simulink model "DC_Charging_Sequence_Block_updated"  (R2024b)
settings: Solver=FixedStepDiscrete  StartTime=0.0  StopTime=10.0  FixedStep=0.01  RelTol=1e-3
undefined symbols (not defined in the file or in its folder): CCM, raptor_get_safe_string, raptor_xcp_function
libraries: Raptor_lib x28
settings Model: RaptorUIDSize=4  Raptor_Target=CCM-58NN-112-2403  Raptor_Calloc=NonVolatile (EEPROM)  Raptor_ecuaddr=11  RaptorBuildNum=-1  Creator=noahm  LastModifiedBy=malul
settings OptimizationCC: DefaultParameterBehavior=Inlined  UseSpecifiedMinMax=on  InlineInvariantSignals=on  EnhancedBackFolding=on  PassReuseOutputArgsAs=Individual arguments  InitFltsAndDblsToZero=on  NoFixptDivByZeroProtection=on  EfficientFloat2IntCast=on  OptimizeBlockOrder=speed  DifferentSizesBufferReuse=on  OptimizationCustomize=off  EfficientTunableParamExpr=on
settings DebuggingCC: UnderspecifiedInitializationDetection=Classic  MergeDetectMultiDrivingBlocksExec=none  InheritedTsInSrcMsg=none  ParameterTunabilityLossMsg=error
settings HardwareCC: TargetIntDivRoundTo=Zero  TargetEndianess=BigEndian  ProdEqTarget=off
settings ModelReferenceCC: PropagateSignalLabelsOutOfModel=off
settings SFSimCC: MATLABDynamicMemAlloc=off
settings RTWCC: Description=Raptor (tm)  SystemTargetFile=raptor.tlc  MakeCommand=raptor_make_rtw  TemplateMakefile=raptor_tmf
settings CodeAppCC: ForceParamTrailComments=on  IgnoreCustomStorageClasses=off  MaxIdLength=100  OperatorAnnotations=on  SimulinkDataObjDesc=on  SFDataObjDesc=on  InsertBlockDesc=on
settings STFCustomTargetCC: TargetLangStandard=C99 (ISO)  MultiwordLength=256  GenerateSampleERTMain=on  CombineOutputUpdateFcns=on  CombineSignalStateStructs=on  ERTCustomFileBanners=on  SupportComplex=off  SupportContinuousTime=off  SupportNonInlinedSFcns=off  RemoveResetFunc=on  MATLABClassNameForMDSCustomization=Simulink.SoftwareTarget.ERTCustomization  SystemTargetFile=raptor.tlc
settings ERTTargetCC: TargetLangStandard=C99 (ISO)  GenerateSampleERTMain=on  ParMdlRefBuildCompliant=off  CompOptLevelCompliant=off  ConcurrentExecutionCompliant=off  CombineSignalStateStructs=on  SupportComplex=off  ModelStepFunctionPrototypeControlCompliant=off  CPPClassGenCompliant=off  UseToolchainInfoCompliant=off  ERTCustomFileTemplate=example_file_process.tlc

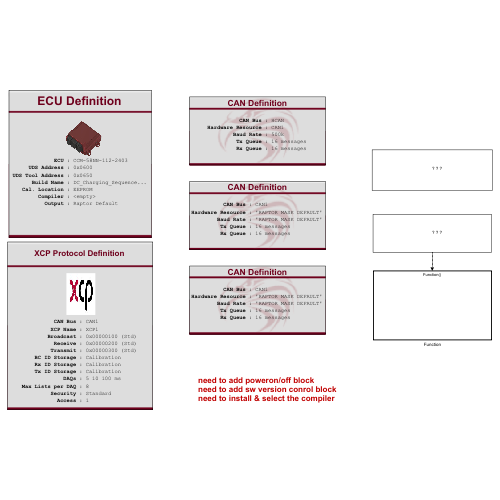
[thumbnail: Simulink's stored preview of the top-level diagram]
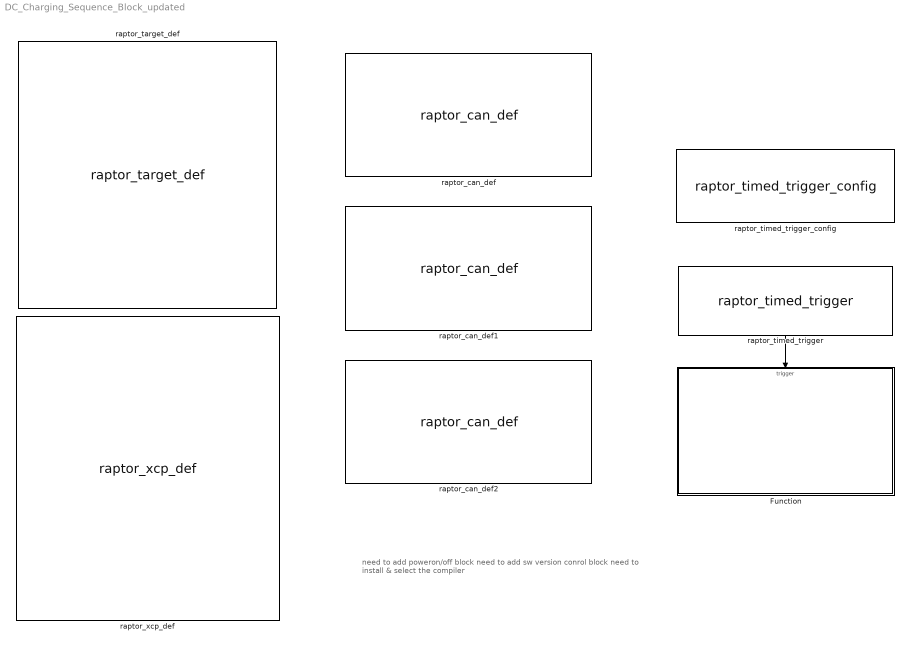
== system DC_Charging_Sequence_Block_updated ==
  note: need to add poweron/off block
      | need to add sw version conrol block
      | need to install & select the compiler
  Function : Subsystem
  raptor_can_def : Raptor_lib/CAN/raptor_can_def  canBus='HCAN'  resourceValues=CAN1|CAN2|CAN3|CAN4|CAN5|CAN6|CAN7|CAN8|(None)  resource=CAN1  baudRateValues=33k|50k|100k|125k|200k|250k|333k|500k|667k|800k|1000k  baudRate=500k  useCustomBR=0  customBR='CustomBaudRate'  enable_baud_rate_config=0  sim_func_name='ConfigureCANBaudRate'  createButton=0  updateButton=0  txQueueSize=16  rxQueueSize=16
      settings: SourceProductName=Raptor
  raptor_can_def1 : Raptor_lib/CAN/raptor_can_def  canBus='CAN1'  resourceValues=CAN1|CAN2|CAN3|CAN4|CAN5|CAN6|CAN7|CAN8|(None)  resource='RAPTOR MASK DEFAULT'  baudRateValues=(None)  baudRate='RAPTOR MASK DEFAULT'  useCustomBR=0  customBR='CustomBaudRate'  enable_baud_rate_config=0  sim_func_name='ConfigureCANBaudRate'  createButton=[]  updateButton=[]  txQueueSize=16  rxQueueSize=16
      settings: SourceProductName=Raptor
  raptor_can_def2 : Raptor_lib/CAN/raptor_can_def  canBus='CAN1'  resourceValues=CAN1|CAN2|CAN3|CAN4|CAN5|CAN6|CAN7|CAN8|(None)  resource='RAPTOR MASK DEFAULT'  baudRateValues=(None)  baudRate='RAPTOR MASK DEFAULT'  useCustomBR=0  customBR='CustomBaudRate'  enable_baud_rate_config=0  sim_func_name='ConfigureCANBaudRate'  createButton=[]  updateButton=[]  txQueueSize=16  rxQueueSize=16
      settings: SourceProductName=Raptor
  raptor_target_def : Raptor_lib/Configuration/raptor_target_def  targetValues=CCM-58NN-112-2403|CCM-TC377-112-2403|DISP-VC128-1901|DISP-VC320L-1402|DISP-VC320-1204|DISP-VC800-1402|DISP-VC500-1904|DISP-VC700-2003|DISP-VC300R-2004|GCM-5634M-070-1559|GCM-5634M-070-1562|EOL-58NN-176-2204|ECM-1793-196-1503|GCM-1793-196-1503|GCM-5605B-048-1906|GCM-5605B-048-2104|RCM-5743R-080-2203|RCM-5743R-080-2304|UAS-5743R-047-2102|UAS-5743R-047-2107|RCM-58NN-112-2103|RCM-58NN-112-2202|RCM-58NN-112-2208|RCM-58NN-112-2410|GCM-TC234-044-2409|GCM-TC277-106-2407|GCM-TC277-108-2406|GCM-TC337-056-2402|GCM-TC367-111-2301|HCM-5604-036-1303|HCM-5604-036-1702  target=CCM-58NN-112-2403  simpack=0  simulator=0  heap=2*1024  stack=4*1024  fgndStack=2*1024  bgndStack=2*1024  idleStack=1024  intStack=1536  sdStack=1024  appStack=1024  ecuaddr=11  uds_server_addr_ext=0  uds_server_addr=hex2dec('600')  uds_client_addr=hex2dec('650')  callocValues=Constant (FLASH)|NonVolatile (EEPROM)  calloc=NonVolatile (EEPROM)  compilerValues=[]  compiler=<empty>  setFileName=0  exeName=[raptor_get_safe_string(bdroot) '_']  addBuildNum=0  minVerChars=3  extraOutput=1  buildLocationValues=Raptor Default|Model Directory|User Defined  buildLocation=Raptor Default  exeLocation=''  exeFileButton=0  a2lLocation=''  a2lFileButton=0  rpgLocation=''  rpgFileButton=0
      settings: SourceProductName=Raptor
  raptor_timed_trigger : Raptor_lib/Triggers/raptor_timed_trigger  triggerValues=[]  trigger=Foreground  inherited=0  alwaysEnabled=1  triggerPriority=0  triggerName=FGND__bznT
      settings: SourceProductName=Raptor
  raptor_timed_trigger_config : Raptor_lib/Triggers/raptor_timed_trigger_config  triggerValues=Foreground|Background  trigger=Foreground  period=10
      settings: SourceProductName=Raptor
  raptor_xcp_def : Raptor_lib/Configuration/raptor_xcp_def  XCPname='XCP1'  canBus='CAN1'  bcID=hex2dec('100')  bcID_TypeValues=[]  bcID_Type=Standard  rxID=hex2dec('200')  rxID_TypeValues=[]  rxID_Type=Standard  txID=hex2dec('300')  txID_TypeValues=[]  txID_Type=Standard  daqRates=[5 10 100]  numODTs=8  genCANAPE=0  genVISION=0  securityValues=[]  security=Standard  dllName=raptor_XCPSecurity.dll  accessValues=[]  access=1  bcStorageValues=[]  bcStorage=Calibration  txStorageValues=[]  txStorage=Calibration  rxStorageValues=[]  rxStorage=Calibration
      settings: SourceProductName=Raptor
  wires:
  raptor_timed_trigger/1 -> Function/Trigger

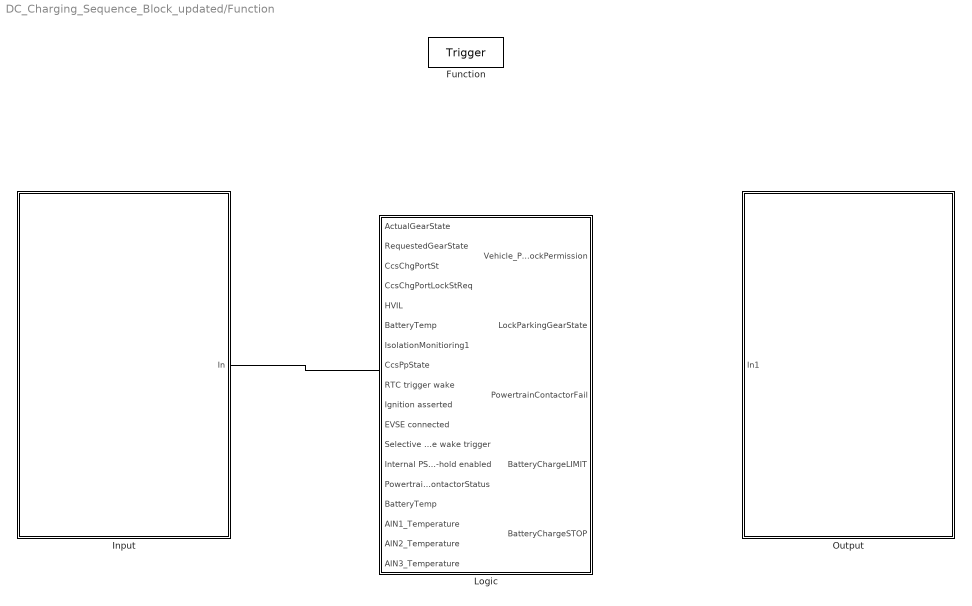
== system DC_Charging_Sequence_Block_updated/Function ==
  Function : TriggerPort  TriggerType=function-call  VariantControl=(inherit)  PortDimensions=1
  Input : Subsystem
  Logic : Subsystem
  Output : Subsystem
  wires:
  Input/1(In) -> ?
  ? -> Output/1(In1)

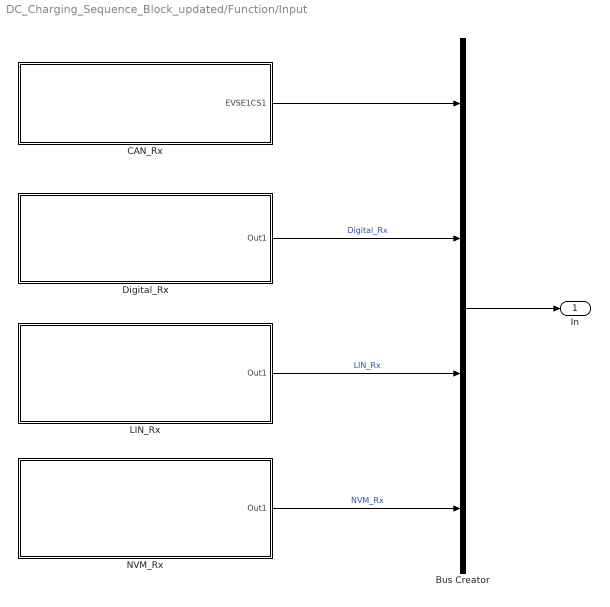
== system DC_Charging_Sequence_Block_updated/Function/Input ==
  Bus Creator : BusCreator  Inputs=4
  CAN_Rx : Subsystem
  Digital_Rx : Subsystem
  LIN_Rx : Subsystem
  NVM_Rx : Subsystem
  In : Outport
  wires:
  Digital_Rx/1(Out1) -> Bus Creator/2  "Digital_Rx"
  LIN_Rx/1(Out1) -> Bus Creator/3  "LIN_Rx"
  NVM_Rx/1(Out1) -> Bus Creator/4  "NVM_Rx"
  Bus Creator/1 -> In/1
  CAN_Rx/1(EVSE1CS1) -> Bus Creator/1

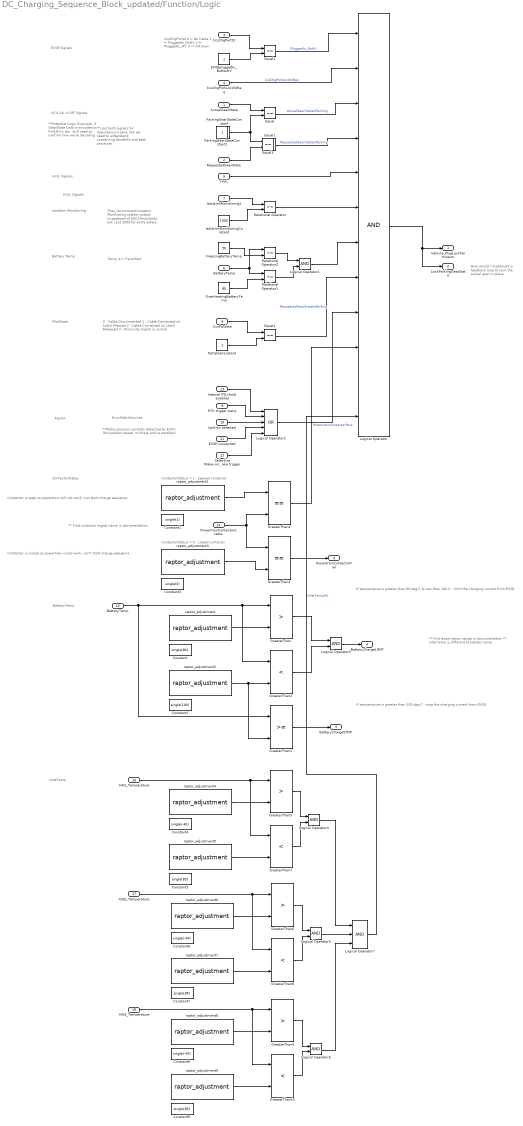
== system DC_Charging_Sequence_Block_updated/Function/Logic ==
  note: ContactorStatus
  note: EVSE Signals
  note: VCU Car is Off Signals
  note: How would I implement a feedback loop to lock the actual gear in place.
  note: **Potential Logic Example, if GearState Data is encoded as P=0,R=1, etc.
      | Still need to confirm how we're decoding
  note: **I put both signals for redundancy's sake, but we need to understand conserving bandwith and best practices.
  note: CcsChgPortst
      | 0 = No Cable
      | 1 = PluggedIn_NoHV
      | 2 = PluggedIn_HV
      | 3 = Unknown
  note: HVIL Signals
  note: Isolation Monitioring
  note: They recommend Isolation Monitioring system output Impedance of 500 Ohms/Volts, but I put 1000 for extra safety.
  note: Temp is in Farenheit
  note: Battery Temp
  note: PilotState
  note: 0 - Cable Disconnected
      | 1 - Cable Connected w/ Latch Pressed
      | 2 - Cable Connected w/ Latch Released
      | 3 - Proximity Signal is invalid
  note: HVIL Signals
  note: KeyOn
  note: **Wake sources currently detected by EVCC (bit position based, multiple active possible)
  note: EvccWakeSources
  note: Contactor is open so powertrain will not work, can start charge sequence
  note: Contactor is closed so powertrain could work, can't start charge sequence
  note: ContactorStatus = 1 : opened contactor
  note: ** Find contactor signal name in documentation
  note: ContactorStatus = 0 : closed contactor
  note: If temperature is greater than 100 deg C - stop the charging current from EVSE
  note: ** Find exact temp values in documentation
      | ** Inlet temp is different to battery temp
  note: If temperature is greater than 80 deg C & less than 100 C - limit the charging current from EVSE
  note: BatteryTemp
  note: InletTemp
  ActualGearState : Inport
  RequestedGearState : Inport  Port=2
  CcsChgPortSt : Inport  Port=3
  CcsChgPortLockStReq : Inport  Port=4
  HVIL : Inport  Port=5
  " BatteryTemp" : Inport  Port=6
  IsolationMonitioring1 : Inport  Port=7
  CcsPpState : Inport  Port=8
  RTC trigger wake : Inport  Port=9
  Ignition asserted : Inport  Port=10
  EVSE connected : Inport  Port=11
  Selective Wake-on-CAN message wake trigger : Inport  Port=12
  Internal PSU-hold enabled : Inport  Port=13
  PowertrainContactorStatus : Inport  Port=14
  BatteryTemp : Inport  Port=15
  AIN1_Temperature : Inport  Port=16
  "AIN2_Temperature " : Inport  Port=17
  AIN3_Temperature : Inport  Port=18
  Constant : Constant  Value=single(80)
  Constant1 : Constant  Value=single(1)
  Constant2 : Constant  Value=single(100)
  Constant3 : Constant  Value=single(0)
  Constant4 : Constant  Value=single(-40)
  Constant5 : Constant  Value=single(85)
  Constant6 : Constant  Value=single(-40)
  Constant7 : Constant  Value=single(85)
  Constant8 : Constant  Value=single(-40)
  Constant9 : Constant  Value=single(85)
  EVSEpluggedIn_ButNoHV : Constant
  Equal{,1..4} (5 alike) : RelationalOperator  Operator===  OutDataTypeStr=boolean  RndMeth=Simplest  InputSameDT=off
  FreezingBatteryTemp : Constant  Value=50
  GreaterThan{,5..6,9} (4 alike) : RelationalOperator  Operator=>  OutDataTypeStr=boolean  RndMeth=Simplest  InputSameDT=off
  GreaterThan1 : RelationalOperator  OutDataTypeStr=boolean  RndMeth=Simplest  InputSameDT=off
  GreaterThan{2,7..8,10} (4 alike) : RelationalOperator  Operator=<  OutDataTypeStr=boolean  RndMeth=Simplest  InputSameDT=off
  GreaterThan3 : RelationalOperator  Operator===  OutDataTypeStr=boolean  RndMeth=Simplest  InputSameDT=off
  GreaterThan4 : RelationalOperator  Operator===  OutDataTypeStr=boolean  RndMeth=Simplest  InputSameDT=off
  IsolationMonitioringConstant : Constant  Value=1000
  Logical Operator : Logic  Inputs=12  AllPortsSameDT=off  OutDataTypeStr=boolean
  Logical Operator{1,3..6} (5 alike) : Logic  AllPortsSameDT=off  OutDataTypeStr=boolean
  Logical Operator2 : Logic  Operator=OR  Inputs=5  AllPortsSameDT=off  OutDataTypeStr=boolean
  Logical Operator7 : Logic  Inputs=3  AllPortsSameDT=off  OutDataTypeStr=boolean
  OverHeatingBatteryTemp : Constant  Value=80
  ParkingGearStateConstant : Constant
  ParkingGearStateConstant1 : Constant
  PpCableConstant : Constant
  Relational Operator : RelationalOperator  OutDataTypeStr=boolean  RndMeth=Simplest  InputSameDT=off
  Relational Operator1 : RelationalOperator  Operator=<=  OutDataTypeStr=boolean  RndMeth=Simplest  InputSameDT=off
  Relational Operator2 : RelationalOperator  OutDataTypeStr=boolean  RndMeth=Simplest  InputSameDT=off
  raptor_adjustment : Raptor_lib/Data Storage/raptor_adjustment  paramName='TempThresholdLimit1'  nameSource=Parameter  initValue=80  dataType=single  storage=Calibration  calDispType=Number  calEnum={'False', 'True'}  calGain=1.0  calOffset=0.0  calMax=inf  calMin=-inf  calFormat='-1'  calUnit=''  calHelp=''  calAccess=1  calFunction=raptor_xcp_function(gcb)  calDispHeaders=off  calColHeaders={'Col1' 'Col2' 'Col3'}  calRowHeaders={'Row1' 'Row2' 'Row3'}
      settings: SourceProductName=Raptor
  raptor_adjustment1 : Raptor_lib/Data Storage/raptor_adjustment  paramName='ContactorStatus1'  nameSource=Parameter  initValue=1  dataType=single  storage=Calibration  calDispType=Number  calEnum={'False', 'True'}  calGain=1.0  calOffset=0.0  calMax=inf  calMin=-inf  calFormat='-1'  calUnit=''  calHelp=''  calAccess=1  calFunction=raptor_xcp_function(gcb)  calDispHeaders=off  calColHeaders={'Col1' 'Col2' 'Col3'}  calRowHeaders={'Row1' 'Row2' 'Row3'}
      settings: SourceProductName=Raptor
  raptor_adjustment2 : Raptor_lib/Data Storage/raptor_adjustment  paramName='TempThresholdLimit2'  nameSource=Parameter  initValue=100  dataType=single  storage=Calibration  calDispType=Number  calEnum={'False', 'True'}  calGain=1.0  calOffset=0.0  calMax=inf  calMin=-inf  calFormat='-1'  calUnit=''  calHelp=''  calAccess=1  calFunction=raptor_xcp_function(gcb)  calDispHeaders=off  calColHeaders={'Col1' 'Col2' 'Col3'}  calRowHeaders={'Row1' 'Row2' 'Row3'}
      settings: SourceProductName=Raptor
  raptor_adjustment3 : Raptor_lib/Data Storage/raptor_adjustment  paramName='ContactorStatus0'  nameSource=Parameter  initValue=0  dataType=single  storage=Calibration  calDispType=Number  calEnum={'False', 'True'}  calGain=1.0  calOffset=0.0  calMax=inf  calMin=-inf  calFormat='-1'  calUnit=''  calHelp=''  calAccess=1  calFunction=raptor_xcp_function(gcb)  calDispHeaders=off  calColHeaders={'Col1' 'Col2' 'Col3'}  calRowHeaders={'Row1' 'Row2' 'Row3'}
      settings: SourceProductName=Raptor
  raptor_adjustment4 : Raptor_lib/Data Storage/raptor_adjustment  paramName='InletMinTempThreshold'  nameSource=Parameter  initValue=-40  dataType=single  storage=Calibration  calDispType=Number  calEnum={'False', 'True'}  calGain=1.0  calOffset=0.0  calMax=inf  calMin=-inf  calFormat='-1'  calUnit=''  calHelp=''  calAccess=1  calFunction=raptor_xcp_function(gcb)  calDispHeaders=off  calColHeaders={'Col1' 'Col2' 'Col3'}  calRowHeaders={'Row1' 'Row2' 'Row3'}
      settings: SourceProductName=Raptor
  raptor_adjustment5 : Raptor_lib/Data Storage/raptor_adjustment  paramName='InletMaxTempThreshold'  nameSource=Parameter  initValue=85  dataType=single  storage=Calibration  calDispType=Number  calEnum={'False', 'True'}  calGain=1.0  calOffset=0.0  calMax=inf  calMin=-inf  calFormat='-1'  calUnit=''  calHelp=''  calAccess=1  calFunction=raptor_xcp_function(gcb)  calDispHeaders=off  calColHeaders={'Col1' 'Col2' 'Col3'}  calRowHeaders={'Row1' 'Row2' 'Row3'}
      settings: SourceProductName=Raptor
  raptor_adjustment6 : Raptor_lib/Data Storage/raptor_adjustment  paramName='InletMinTempThreshold'  nameSource=Parameter  initValue=-40  dataType=single  storage=Calibration  calDispType=Number  calEnum={'False', 'True'}  calGain=1.0  calOffset=0.0  calMax=inf  calMin=-inf  calFormat='-1'  calUnit=''  calHelp=''  calAccess=1  calFunction=raptor_xcp_function(gcb)  calDispHeaders=off  calColHeaders={'Col1' 'Col2' 'Col3'}  calRowHeaders={'Row1' 'Row2' 'Row3'}
      settings: SourceProductName=Raptor
  raptor_adjustment7 : Raptor_lib/Data Storage/raptor_adjustment  paramName='InletMaxTempThreshold'  nameSource=Parameter  initValue=85  dataType=single  storage=Calibration  calDispType=Number  calEnum={'False', 'True'}  calGain=1.0  calOffset=0.0  calMax=inf  calMin=-inf  calFormat='-1'  calUnit=''  calHelp=''  calAccess=1  calFunction=raptor_xcp_function(gcb)  calDispHeaders=off  calColHeaders={'Col1' 'Col2' 'Col3'}  calRowHeaders={'Row1' 'Row2' 'Row3'}
      settings: SourceProductName=Raptor
  raptor_adjustment8 : Raptor_lib/Data Storage/raptor_adjustment  paramName='InletMinTempThreshold'  nameSource=Parameter  initValue=-40  dataType=single  storage=Calibration  calDispType=Number  calEnum={'False', 'True'}  calGain=1.0  calOffset=0.0  calMax=inf  calMin=-inf  calFormat='-1'  calUnit=''  calHelp=''  calAccess=1  calFunction=raptor_xcp_function(gcb)  calDispHeaders=off  calColHeaders={'Col1' 'Col2' 'Col3'}  calRowHeaders={'Row1' 'Row2' 'Row3'}
      settings: SourceProductName=Raptor
  raptor_adjustment9 : Raptor_lib/Data Storage/raptor_adjustment  paramName='InletMaxTempThreshold'  nameSource=Parameter  initValue=85  dataType=single  storage=Calibration  calDispType=Number  calEnum={'False', 'True'}  calGain=1.0  calOffset=0.0  calMax=inf  calMin=-inf  calFormat='-1'  calUnit=''  calHelp=''  calAccess=1  calFunction=raptor_xcp_function(gcb)  calDispHeaders=off  calColHeaders={'Col1' 'Col2' 'Col3'}  calRowHeaders={'Row1' 'Row2' 'Row3'}
      settings: SourceProductName=Raptor
  Vehicle_PlugLockPermission : Outport
  LockParkingGearState : Outport  Port=2
  PowertrainContactorFail : Outport  Port=3
  BatteryChargeLIMIT : Outport  Port=4
  BatteryChargeSTOP : Outport  Port=5
  wires:
  Logical Operator/1 -> LockParkingGearState/1, Vehicle_PlugLockPermission/1
  ActualGearState/1 -> Equal/1
  ParkingGearStateConstant/1 -> Equal1/1, Equal/2
  Equal/1 -> Logical Operator/3  "ActualGearStateIsParking"
  RequestedGearState/1 -> Equal1/2
  Equal1/1 -> Logical Operator/4  "RequestedGearStateIsParking"
  EVSEpluggedIn_ButNoHV/1 -> Equal2/2
  CcsChgPortSt/1 -> Equal2/1
  Equal2/1 -> Logical Operator/1  "PluggedIn_NoHV"
  CcsChgPortLockStReq/1 -> Logical Operator/2  "CcsChgPortLockStReq"
  HVIL/1 -> Logical Operator/5
  IsolationMonitioringConstant/1 -> Relational Operator/2
  Relational Operator/1 -> Logical Operator/6
  IsolationMonitioring1/1 -> Relational Operator/1
  " BatteryTemp"/1 -> Relational Operator2/1, Relational Operator1/1
  OverHeatingBatteryTemp/1 -> Relational Operator1/2
  FreezingBatteryTemp/1 -> Relational Operator2/2
  Relational Operator2/1 -> Logical Operator1/1
  Relational Operator1/1 -> Logical Operator1/2
  Logical Operator1/1 -> Logical Operator/7
  CcsPpState/1 -> Equal4/1
  PpCableConstant/1 -> Equal4/2
  Equal4/1 -> Logical Operator/8  "RequestedGearStateIsParking"
  Logical Operator2/1 -> Logical Operator/9
  Internal PSU-hold enabled/1 -> Logical Operator2/1
  RTC trigger wake/1 -> Logical Operator2/2
  Ignition asserted/1 -> Logical Operator2/3
  EVSE connected/1 -> Logical Operator2/4
  Selective Wake-on-CAN message wake trigger/1 -> Logical Operator2/5
  PowertrainContactorStatus/1 -> GreaterThan3/1, GreaterThan4/2
  raptor_adjustment1/1 -> GreaterThan4/1
  GreaterThan3/1 -> PowertrainContactorFail/1
  raptor_adjustment3/1 -> GreaterThan3/2
  GreaterThan4/1 -> Logical Operator/10  "PowertrainContactorPass"
  raptor_adjustment/1 -> GreaterThan/2
  BatteryTemp/1 -> GreaterThan1/1, GreaterThan2/1, GreaterThan/1
  raptor_adjustment2/1 -> GreaterThan1/2, GreaterThan2/2
  GreaterThan2/1 -> Logical Operator3/2
  GreaterThan1/1 -> BatteryChargeSTOP/1
  Logical Operator3/1 -> BatteryChargeLIMIT/1
  GreaterThan/1 -> Logical Operator3/1
  raptor_adjustment5/1 -> GreaterThan7/2
  AIN3_Temperature/1 -> GreaterThan10/1, GreaterThan9/1
  raptor_adjustment8/1 -> GreaterThan9/2
  AIN1_Temperature/1 -> GreaterThan7/1, GreaterThan5/1
  Logical Operator6/1 -> Logical Operator7/3
  GreaterThan5/1 -> Logical Operator4/1
  raptor_adjustment9/1 -> GreaterThan10/2
  raptor_adjustment4/1 -> GreaterThan5/2
  raptor_adjustment6/1 -> GreaterThan6/2
  GreaterThan9/1 -> Logical Operator6/1
  "AIN2_Temperature "/1 -> GreaterThan8/1, GreaterThan6/1
  raptor_adjustment7/1 -> GreaterThan8/2
  GreaterThan6/1 -> Logical Operator5/1
  GreaterThan10/1 -> Logical Operator6/2
  Logical Operator5/1 -> Logical Operator7/2
  GreaterThan7/1 -> Logical Operator4/2
  Logical Operator4/1 -> Logical Operator7/1
  GreaterThan8/1 -> Logical Operator5/2
  Logical Operator7/1 -> Logical Operator/12  "InletTempOK"

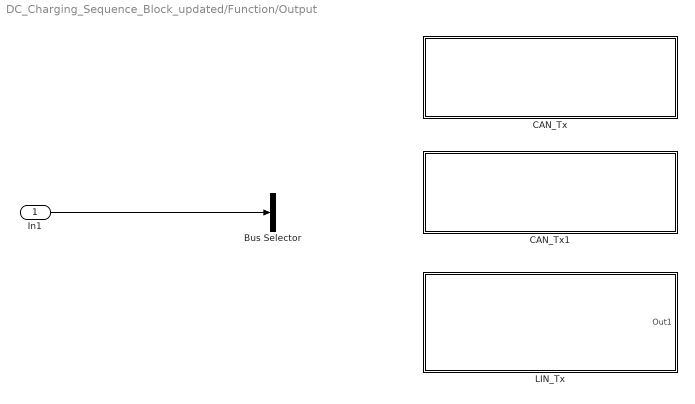
== system DC_Charging_Sequence_Block_updated/Function/Output ==
  In1 : Inport
  Bus Selector : BusSelector  OutputSignals=signal1,signal2
  CAN_Tx : Subsystem
  CAN_Tx1 : Subsystem
  LIN_Tx : Subsystem
  wires:
  In1/1 -> Bus Selector/1

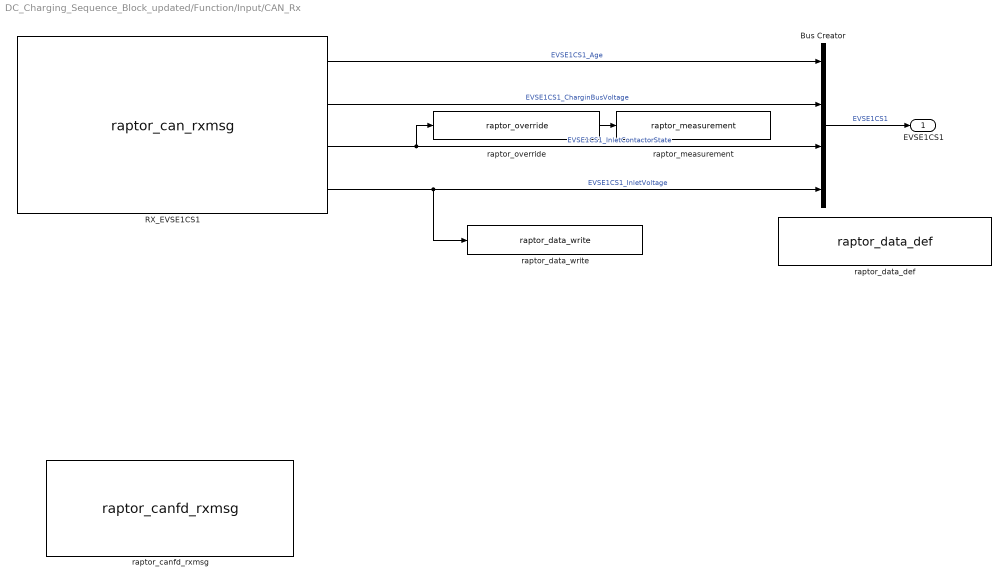
== system DC_Charging_Sequence_Block_updated/Function/Input/CAN_Rx ==
  Bus Creator : BusCreator  Inputs=4
  RX_EVSE1CS1 : Raptor_lib/CAN/raptor_can_rxmsg  canDefinition=struct('dbcFile', 'CCU_VehicleInterface_R5371.dbc','message', 'EVSE1CS1','comment', '','signals', {{'ChargingBusVoltage','InletContactorState','InletVoltage'}},'enabled', [ 1 1 1;],'scaled', [ 1 1 1;],'canBus', '''CAN1''','messageID', [ 419084891;],'idMask', [ 536870911;],'payloadMask', [],'payloadValue', [],'period', [ 0;],'mailbox', '''''','queueSize', [ 1;],'label', [ 0;],'ver', [ 2;],'showID', [ 0;],'showRaw', [ 0;],'showRawMsg', [ 0;],'useStartVals', [ 0;],'extendedId', [ 1;],'showAge', [ 1;],'useSimFunc', [ 0;],'sim_func_name', '''''','fill', [ 0;],'editID', [ 0;],'signalOrder', [ 1;],'signalAscDes', [ 1;],'msgLength', [ 8;])  canBus='CAN1'  mailbox=''  payloadMask=[]  payloadValue=[]  idMask=hex2dec('1FFFFFFF')  queueSize=1  showID=0  label=0  fill=0  id=419084891  showRaw=0  showAge=1  signalOrder=1  signalInfo={{struct('Name', 'ChargingBusVoltage','StartBit', [ 16;],'SignalSize', [ 16;],'ByteOrder', 'LittleEndian','ValueType', 'Integer','Class', 'uint16','Signed', '0','Factor', [ 0.05;],'Offset', [ 0;],'Min', [ 0;],'Max', [ 3276.75;],'Units', 'V','Comment', 'notused[SPN_13180]','Multiplexor', [ 0;],'Multiplexed', [ 0;],'Muxor_Name', '','MultiplexMode_Min', [],'MultiplexMode_Max', [],'StartVal', [ 0;]),struct('Name', 'InletContactorState','StartBit', [ 32;],'SignalSize', [ 2;],'ByteOrder', 'LittleEndian','ValueType', 'Integer','Class', 'uint8','Signed', '0','Factor', [ 1;],'Offset', [ 0;],'Min', [ 0;],'Max', [ 3;],'Units', 'enum','Comment', 'dbc[SPN_13181]','Multiplexor', [ 0;],'Multiplexed', [ 0;],'Muxor_Name', '','MultiplexMode_Min', [],'MultiplexMode_Max', [],'StartVal', [ 0;]),struct('Name', 'InletVoltage','StartBit', [ 0;],'SignalSize', [ 16;],'ByteOrder', 'LittleEndian','ValueType', 'Integer','Class', 'uint16','Signed', '0','Factor', [ 0.05;],'Offset', [ 0;],'Min', [ 0;],'Max', [ 3276.75;],'Units', 'V','Comment', 'dbc[SPN_13179]','Multiplexor', [ 0;],'Multiplexed', [ 0;],'Muxor_Name', '','MultiplexMode_Min', [],'MultiplexMode_Max', [],'StartVal', [ 0;])}}  showRawMsg=0  useSimFunc=0  sim_func_name=''  useStartVals=0  extendedId=1
      settings: SourceProductName=Raptor
  raptor_canfd_rxmsg : Raptor_lib/CAN/raptor_canfd_rxmsg  canDefinition=struct('dbcFile', 'can_example.dbc','message', 'ExampleMsgTxExtended','comment', 'Example message','signals', {{'Enable','EngineSpeed','EngineTemperature'}},'enabled', [ 1 1 1;],'scaled', [ 1 1 1;],'canBus', '''CAN1''','messageID', [ 777;],'idMask', [ 536870911;],'payloadMask', [],'payloadValue', [],'period', [ 0;],'mailbox', '''''','queueSize', [ 1;],'label', [ 0;],'ver', [ 2;],'showID', [ 0;],'showRaw', [ 0;],'showRawMsg', [ 0;],'showAge', [ 1;],'useSimFunc', [ 0;],'sim_func_name', '''''','enableBRS', [ 0;],'fill', [ 0;],'editID', [ 0;],'signalOrder', [ 1;],'signalAscDes', [ 1;],'msgLength', [ 8;])  canBus='CAN1'  mailbox=''  payloadMask=[]  payloadValue=[]  idMask=hex2dec('1FFFFFFF')  queueSize=1  showID=0  label=0  fill=0  id=777  showRaw=0  showAge=1  signalOrder=1  signalInfo={{struct('Name', 'Enable','StartBit', [ 0;],'SignalSize', [ 1;],'ByteOrder', 'BigEndian','ValueType', 'UNSIGNED','Class', 'uint8','Signed', [ 0;],'Factor', [ 1;],'Offset', [ 0;],'Min', [ 0;],'Max', [ 1;],'Units', '','StartVal', [ 0;],'Comment', '','Multiplexed', [ 0;],'Multiplexor', [ 0;],'MultiplexMode_Min', [],'MultiplexMode_Max', []),struct('Name', 'EngineSpeed','StartBit', [ 16;],'SignalSize', [ 16;],'ByteOrder', 'BigEndian','ValueType', 'UNSIGNED','Class', 'uint16','Signed', [ 0;],'Factor', [ 0.1;],'Offset', [ 0;],'Min', [ 0;],'Max', [ 6500;],'Units', 'rpm','StartVal', [ 0;],'Comment', '','Multiplexed', [ 0;],'Multiplexor', [ 0;],'MultiplexMode_Min', [],'MultiplexMode_Max', []),struct('Name', 'EngineTemperature','StartBit', [ 32;],'SignalSize', [ 16;],'ByteOrder', 'BigEndian','ValueType', 'UNSIGNED','Class', 'uint16','Signed', [ 0;],'Factor', [ 0.01;],'Offset', [ -40;],'Min', [ -40;],'Max', [ 500;],'Units', 'degC','StartVal', [ 0;],'Comment', '','Multiplexed', [ 0;],'Multiplexor', [ 0;],'MultiplexMode_Min', [],'MultiplexMode_Max', [])}}  showRawMsg=0  useSimFunc=0  sim_func_name=''  useStartVals=0  showFD=0  fdEnable=0  showBRS=0  brsEnable=0  extendedId=1
      settings: SourceProductName=Raptor
  raptor_data_def : Raptor_lib/Data Storage/raptor_data_def  dataName='EVSE_InletVoltage'  initValue=0  dataType=single  storage=Volatile (RAM)  calVisible=on  calType=Measurement  calDispType=Number  calEnum={'False', 'True'}  calGain=1.0  calOffset=0  calMin=-inf  calMax=inf  calFormat='-1'  calUnit=''  calHelp=''  calAccess=1  calFunction=raptor_xcp_function(gcb)  calDispHeaders=off  calColHeaders={'Col1' 'Col2' 'Col3'}  calRowHeaders={'Row1' 'Row2' 'Row3'}
      settings: SourceProductName=Raptor
  raptor_data_write : Raptor_lib/Data Storage/raptor_data_write  dataName='EVSE_InletVoltage'  dataShape=Scalar  idxSource=Input Port  idxRow=1  idxCol=1
      settings: SourceProductName=Raptor
  raptor_measurement : Raptor_lib/Data Storage/raptor_measurement  paramName='EVSE_Inlet_Contactor_State'  nameSource=Parameter  calDispType=Number  calEnum={'False', 'True'}  calGain=1.0  calOffset=0.0  calMax=inf  calMin=-inf  calFormat='-1'  calUnit=''  calHelp=''  calAccess=1  calFunction=raptor_xcp_function(gcb)  calVisible=on
      settings: SourceProductName=Raptor
  raptor_override : Raptor_lib/Data Storage/raptor_override  paramName='en_EVSE_Inlet_Contactor_State'  nameSource=Parameter  measurement=None  calDispType=Number  calEnum={'False', 'True'}  calGain=1.0  calOffset=0.0  calMax=inf  calMin=-inf  calFormat='-1'  calUnit=''  calHelp=''  calAccess=1  calFunction="[raptor_xcp_function(gcb) '|'  'Override']"
      settings: SourceProductName=Raptor
  EVSE1CS1 : Outport
  wires:
  RX_EVSE1CS1/3 -> raptor_override/1, Bus Creator/3  "EVSE1CS1_InletContactorState"
  raptor_override/1 -> raptor_measurement/1
  Bus Creator/1 -> EVSE1CS1/1  "EVSE1CS1"
  RX_EVSE1CS1/2 -> Bus Creator/2  "EVSE1CS1_CharginBusVoltage"
  RX_EVSE1CS1/4 -> raptor_data_write/1, Bus Creator/4  "EVSE1CS1_InletVoltage"
  RX_EVSE1CS1/1 -> Bus Creator/1  "EVSE1CS1_Age"

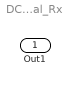
== system DC_Charging_Sequence_Block_updated/Function/Input/Digital_Rx ==
  Out1 : Outport
  wires:
  ? -> Out1/1

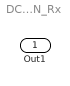
== system DC_Charging_Sequence_Block_updated/Function/Input/LIN_Rx ==
  Out1 : Outport
  wires:
  ? -> Out1/1

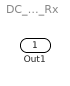
== system DC_Charging_Sequence_Block_updated/Function/Input/NVM_Rx ==
  Out1 : Outport
  wires:
  ? -> Out1/1

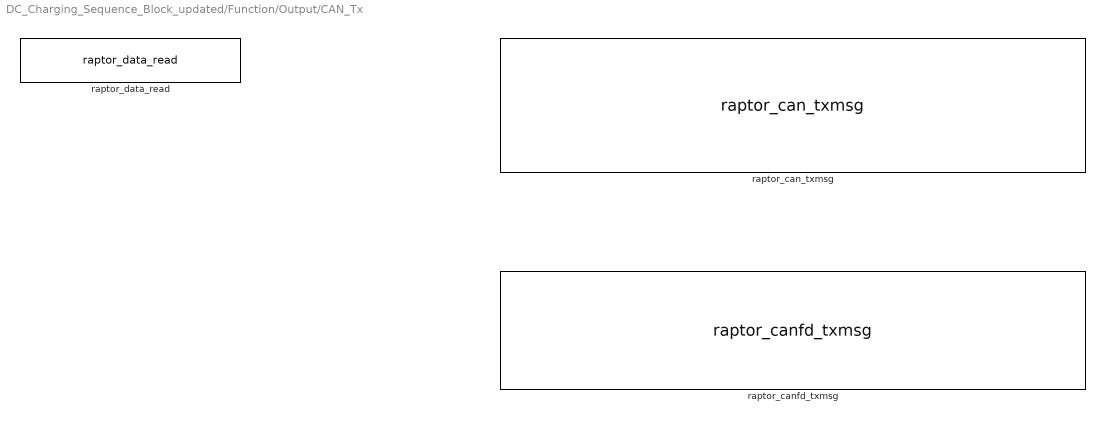
== system DC_Charging_Sequence_Block_updated/Function/Output/CAN_Tx ==
  raptor_can_txmsg : Raptor_lib/CAN/raptor_can_txmsg  canDefinition=struct('dbcFile', '.\CAN\can_example.dbc','message', 'ExampleMsgTxExtended','comment', '','signals', {{'Enable','EngineSpeed','EngineTemperature'}},'enabled', [ 1 1 1;],'canBus', '''CAN1''','messageID', [ 777;],'idMask', [ 536870911;],'payloadMask', [],'payloadValue', [],'period', [ 0;],'mailbox', '','queueSize', [ 1;],'label', [ 0;],'ver', [ 2;],'showID', [ 0;],'showRaw', [ 0;],'fill', [ 0;],'editID', [ 0;],'signalOrder', [ 1;])  canBus='CAN1'  queueSize=1  payloadMask=[]  payloadValue=[]  period=0  showID=0  label=0  idMask=hex2dec('1FFFFFFF')  fill=0  id=777  showRaw=0  signalOrder=1  signalInfo={{struct('Name', 'Enable','StartBit', [ 0;],'SignalSize', [ 1;],'ByteOrder', 'BigEndian','ValueType', 'UNSIGNED','Class', 'uint8','Signed', [ 0;],'Factor', [ 1;],'Offset', [ 0;],'Min', [ 0;],'Max', [ 1;],'Units', '','StartVal', [ 0;],'Comment', '','Multiplexed', [ 0;],'Multiplexor', [ 0;],'MultiplexMode_Min', [],'MultiplexMode_Max', []),struct('Name', 'EngineSpeed','StartBit', [ 16;],'SignalSize', [ 16;],'ByteOrder', 'BigEndian','ValueType', 'UNSIGNED','Class', 'uint16','Signed', [ 0;],'Factor', [ 0.1;],'Offset', [ 0;],'Min', [ 0;],'Max', [ 6500;],'Units', 'rpm','StartVal', [ 0;],'Comment', '','Multiplexed', [ 0;],'Multiplexor', [ 0;],'MultiplexMode_Min', [],'MultiplexMode_Max', []),struct('Name', 'EngineTemperature','StartBit', [ 32;],'SignalSize', [ 16;],'ByteOrder', 'BigEndian','ValueType', 'UNSIGNED','Class', 'uint16','Signed', [ 0;],'Factor', [ 0.01;],'Offset', [ -40;],'Min', [ -40;],'Max', [ 500;],'Units', 'degC','StartVal', [ 0;],'Comment', '','Multiplexed', [ 0;],'Multiplexor', [ 0;],'MultiplexMode_Min', [],'MultiplexMode_Max', [])}}  useSimFunc=0  sim_func_name=''  useStartVals=0
      settings: SourceProductName=Raptor
  raptor_canfd_txmsg : Raptor_lib/CAN/raptor_canfd_txmsg  canDefinition=struct('dbcFile', '.\CAN\can_example.dbc','message', 'ExampleMsgTxExtended','comment', '','signals', {{'Enable','EngineSpeed','EngineTemperature'}},'enabled', [ 1 1 1;],'canBus', '''CAN1''','messageID', [ 777;],'idMask', [ 536870911;],'payloadMask', [],'payloadValue', [],'period', [ 0;],'mailbox', '','queueSize', [ 1;],'label', [ 0;],'ver', [ 2;],'showID', [ 0;],'showRaw', [ 0;],'fill', [ 0;],'editID', [ 0;],'signalOrder', [ 1;])  canBus='CAN1'  queueSize=1  payloadMask=[]  payloadValue=[]  period=0  showID=0  label=0  idMask=hex2dec('1FFFFFFF')  fill=0  id=777  showRaw=0  signalOrder=1  signalInfo={{struct('Name', 'Enable','StartBit', [ 0;],'SignalSize', [ 1;],'ByteOrder', 'BigEndian','ValueType', 'UNSIGNED','Class', 'uint8','Signed', [ 0;],'Factor', [ 1;],'Offset', [ 0;],'Min', [ 0;],'Max', [ 1;],'Units', '','StartVal', [ 0;],'Comment', '','Multiplexed', [ 0;],'Multiplexor', [ 0;],'MultiplexMode_Min', [],'MultiplexMode_Max', []),struct('Name', 'EngineSpeed','StartBit', [ 16;],'SignalSize', [ 16;],'ByteOrder', 'BigEndian','ValueType', 'UNSIGNED','Class', 'uint16','Signed', [ 0;],'Factor', [ 0.1;],'Offset', [ 0;],'Min', [ 0;],'Max', [ 6500;],'Units', 'rpm','StartVal', [ 0;],'Comment', '','Multiplexed', [ 0;],'Multiplexor', [ 0;],'MultiplexMode_Min', [],'MultiplexMode_Max', []),struct('Name', 'EngineTemperature','StartBit', [ 32;],'SignalSize', [ 16;],'ByteOrder', 'BigEndian','ValueType', 'UNSIGNED','Class', 'uint16','Signed', [ 0;],'Factor', [ 0.01;],'Offset', [ -40;],'Min', [ -40;],'Max', [ 500;],'Units', 'degC','StartVal', [ 0;],'Comment', '','Multiplexed', [ 0;],'Multiplexor', [ 0;],'MultiplexMode_Min', [],'MultiplexMode_Max', [])}}  useSimFunc=0  sim_func_name=''  useStartVals=0  brsEnable=0  fdEnable=false
      settings: SourceProductName=Raptor
  raptor_data_read : Raptor_lib/Data Storage/raptor_data_read  dataName='EVSE_InletVoltage'  dataShape=Scalar  idxSource=Input  idxRow=1  idxCol=1
      settings: SourceProductName=Raptor

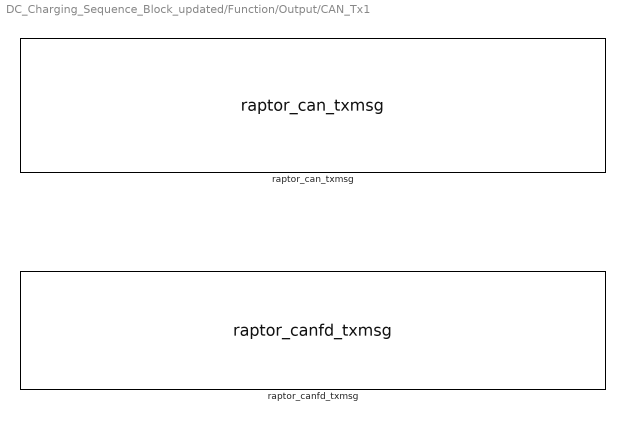
== system DC_Charging_Sequence_Block_updated/Function/Output/CAN_Tx1 ==
  raptor_can_txmsg : Raptor_lib/CAN/raptor_can_txmsg  canDefinition=struct('dbcFile', '.\CAN\can_example.dbc','message', 'ExampleMsgTxExtended','comment', '','signals', {{'Enable','EngineSpeed','EngineTemperature'}},'enabled', [ 1 1 1;],'canBus', '''CAN1''','messageID', [ 777;],'idMask', [ 536870911;],'payloadMask', [],'payloadValue', [],'period', [ 0;],'mailbox', '','queueSize', [ 1;],'label', [ 0;],'ver', [ 2;],'showID', [ 0;],'showRaw', [ 0;],'fill', [ 0;],'editID', [ 0;],'signalOrder', [ 1;])  canBus='CAN1'  queueSize=1  payloadMask=[]  payloadValue=[]  period=0  showID=0  label=0  idMask=hex2dec('1FFFFFFF')  fill=0  id=777  showRaw=0  signalOrder=1  signalInfo={{struct('Name', 'Enable','StartBit', [ 0;],'SignalSize', [ 1;],'ByteOrder', 'BigEndian','ValueType', 'UNSIGNED','Class', 'uint8','Signed', [ 0;],'Factor', [ 1;],'Offset', [ 0;],'Min', [ 0;],'Max', [ 1;],'Units', '','StartVal', [ 0;],'Comment', '','Multiplexed', [ 0;],'Multiplexor', [ 0;],'MultiplexMode_Min', [],'MultiplexMode_Max', []),struct('Name', 'EngineSpeed','StartBit', [ 16;],'SignalSize', [ 16;],'ByteOrder', 'BigEndian','ValueType', 'UNSIGNED','Class', 'uint16','Signed', [ 0;],'Factor', [ 0.1;],'Offset', [ 0;],'Min', [ 0;],'Max', [ 6500;],'Units', 'rpm','StartVal', [ 0;],'Comment', '','Multiplexed', [ 0;],'Multiplexor', [ 0;],'MultiplexMode_Min', [],'MultiplexMode_Max', []),struct('Name', 'EngineTemperature','StartBit', [ 32;],'SignalSize', [ 16;],'ByteOrder', 'BigEndian','ValueType', 'UNSIGNED','Class', 'uint16','Signed', [ 0;],'Factor', [ 0.01;],'Offset', [ -40;],'Min', [ -40;],'Max', [ 500;],'Units', 'degC','StartVal', [ 0;],'Comment', '','Multiplexed', [ 0;],'Multiplexor', [ 0;],'MultiplexMode_Min', [],'MultiplexMode_Max', [])}}  useSimFunc=0  sim_func_name=''  useStartVals=0
      settings: SourceProductName=Raptor
  raptor_canfd_txmsg : Raptor_lib/CAN/raptor_canfd_txmsg  canDefinition=struct('dbcFile', '.\CAN\can_example.dbc','message', 'ExampleMsgTxExtended','comment', '','signals', {{'Enable','EngineSpeed','EngineTemperature'}},'enabled', [ 1 1 1;],'canBus', '''CAN1''','messageID', [ 777;],'idMask', [ 536870911;],'payloadMask', [],'payloadValue', [],'period', [ 0;],'mailbox', '','queueSize', [ 1;],'label', [ 0;],'ver', [ 2;],'showID', [ 0;],'showRaw', [ 0;],'fill', [ 0;],'editID', [ 0;],'signalOrder', [ 1;])  canBus='CAN1'  queueSize=1  payloadMask=[]  payloadValue=[]  period=0  showID=0  label=0  idMask=hex2dec('1FFFFFFF')  fill=0  id=777  showRaw=0  signalOrder=1  signalInfo={{struct('Name', 'Enable','StartBit', [ 0;],'SignalSize', [ 1;],'ByteOrder', 'BigEndian','ValueType', 'UNSIGNED','Class', 'uint8','Signed', [ 0;],'Factor', [ 1;],'Offset', [ 0;],'Min', [ 0;],'Max', [ 1;],'Units', '','StartVal', [ 0;],'Comment', '','Multiplexed', [ 0;],'Multiplexor', [ 0;],'MultiplexMode_Min', [],'MultiplexMode_Max', []),struct('Name', 'EngineSpeed','StartBit', [ 16;],'SignalSize', [ 16;],'ByteOrder', 'BigEndian','ValueType', 'UNSIGNED','Class', 'uint16','Signed', [ 0;],'Factor', [ 0.1;],'Offset', [ 0;],'Min', [ 0;],'Max', [ 6500;],'Units', 'rpm','StartVal', [ 0;],'Comment', '','Multiplexed', [ 0;],'Multiplexor', [ 0;],'MultiplexMode_Min', [],'MultiplexMode_Max', []),struct('Name', 'EngineTemperature','StartBit', [ 32;],'SignalSize', [ 16;],'ByteOrder', 'BigEndian','ValueType', 'UNSIGNED','Class', 'uint16','Signed', [ 0;],'Factor', [ 0.01;],'Offset', [ -40;],'Min', [ -40;],'Max', [ 500;],'Units', 'degC','StartVal', [ 0;],'Comment', '','Multiplexed', [ 0;],'Multiplexor', [ 0;],'MultiplexMode_Min', [],'MultiplexMode_Max', [])}}  useSimFunc=0  sim_func_name=''  useStartVals=0  brsEnable=0  fdEnable=false
      settings: SourceProductName=Raptor

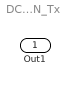
== system DC_Charging_Sequence_Block_updated/Function/Output/LIN_Tx ==
  Out1 : Outport
  wires:
  ? -> Out1/1
